simulink model "main_state_v2"  (R2021b)
settings: Solver=VariableStepAuto  StartTime=0.0  StopTime=10.0  RelTol=1e-3
settings Model: Creator=nose  LastModifiedBy=nose

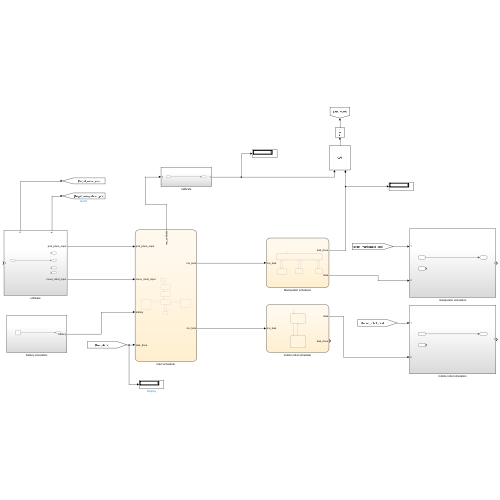
[thumbnail: Simulink's stored preview of the top-level diagram]
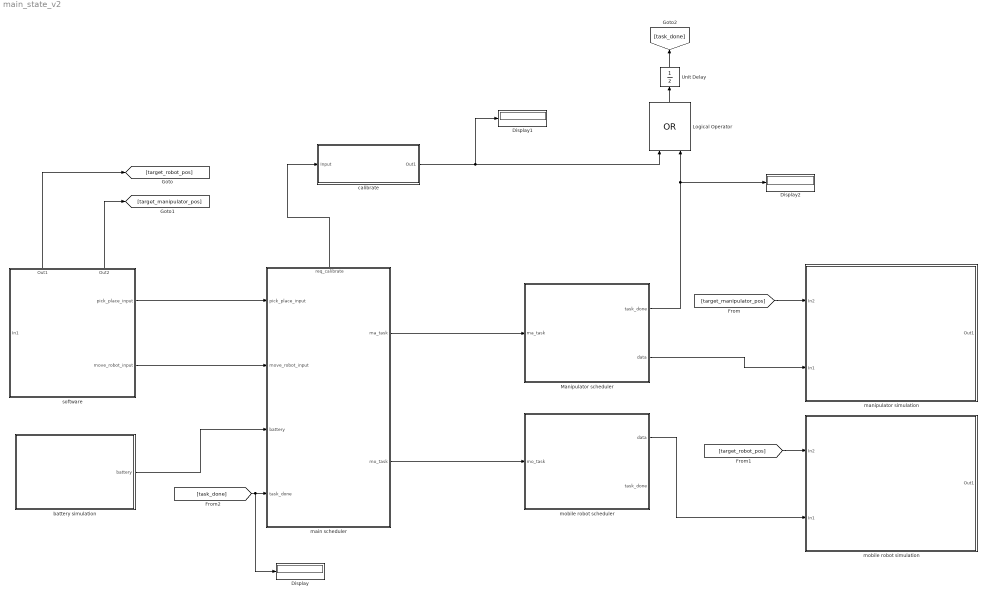
== system main_state_v2 ==
  Display : Display
  Display1 : Display
  Display2 : Display
  Logical Operator : Logic  Operator=OR  AllPortsSameDT=off  OutDataTypeStr=boolean
  Manipulator scheduler : Stateflow chart  TreatAsAtomicUnit=on
  Unit Delay : UnitDelay  SampleTime=-1  HasFrameUpgradeWarning=on
  battery simulation : Subsystem
  calibrate : Subsystem
  main scheduler : Stateflow chart  TreatAsAtomicUnit=on
      settings: PortSchema="{\"entries\":[{\"content\":{\"sides\":[{\"content\":{\"connectorIds\":[\"In1\",\"In4\",\"In2\",\"In3\"]},\"type\":\"ConnectorPlacement.EquallySpacedRectSide\",\"uuid\":\"f5729231-57ab-4499-afbb-6a74bae65d7c\"},{\"content\":{\"connectorIds\":[\"Out2\",\"Out3\"],\"side\":\"RIGHT\"},\"type\":\"ConnectorPlacement.EquallySpacedRectSide\",\"uuid\":\"4bea4fd3-2ca8-4b6f-84e5-251c5021326e\"},{\"content\":{\"connectorIds\":[\"Out1\"],\"side\":\"TOP\"},\"type\":\"ConnectorPlacement.EquallySpacedRectSide\",\"uuid\":\"ba10ffa7-10a0-4e15-a1ab-c6799962567e\"}]},\"type\":\"ConnectorPlacement.EquallySpacedConnector\",\"uuid\":\"fd2ab94f-7982-477b-afda-6ae5ba1f9b27\"}],\"packageUris\":[\"http://schema.mathworks.com/mf0/Connector/R2020b\"],\"version\":\"1.0\"}"
  manipulator simulation : Subsystem
  mobile robot scheduler : Stateflow chart  TreatAsAtomicUnit=on
  mobile robot simulation : Subsystem
  software : Subsystem
      settings: PortSchema="{\"entries\":[{\"content\":{\"sides\":[{\"content\":{\"connectorIds\":[\"In1\"]},\"type\":\"ConnectorPlacement.EquallySpacedRectSide\",\"uuid\":\"68df7bb9-dda6-4834-bc86-6120b81067a6\"},{\"content\":{\"connectorIds\":[\"Out1\",\"Out2\"],\"side\":\"RIGHT\"},\"type\":\"ConnectorPlacement.EquallySpacedRectSide\",\"uuid\":\"97ff30f2-6e8d-41db-be67-1bd246f3902f\"},{\"content\":{\"connectorIds\":[\"Out3\",\"Out4\"],\"side\":\"TOP\"},\"type\":\"ConnectorPlacement.EquallySpacedRectSide\",\"uuid\":\"a9bfe2b4-c08a-4e3f-8415-e43960abb484\"}]},\"type\":\"ConnectorPlacement.EquallySpacedConnector\",\"uuid\":\"6637d52b-a5d0-4863-9f23-94af3600c1a1\"}],\"packageUris\":[\"http://schema.mathworks.com/mf0/Connector/R2020b\"],\"version\":\"1.0\"}"
  wires:
  main scheduler/2(ma_task) -> Manipulator scheduler/1(ma_task)
  main scheduler/3(mo_task) -> mobile robot scheduler/1(mo_task)
  main scheduler/1(req_calibrate) -> calibrate/1(Input)
  battery simulation/1(battery) -> main scheduler/2(battery)
  software/1(pick_place_input) -> main scheduler/1(pick_place_input)
  software/2(move_robot_input) -> main scheduler/4(move_robot_input)
  software/3(Out1) -> [target_robot_pos]
  software/4(Out2) -> [target_manipulator_pos]
  [target_manipulator_pos] -> manipulator simulation/1(In2)
  [target_robot_pos] -> mobile robot simulation/1(In2)
  Manipulator scheduler/2(data) -> manipulator simulation/2(In1)
  mobile robot scheduler/1(data) -> mobile robot simulation/2(In1)
  [task_done] -> Display/1, main scheduler/3(task_done)
  calibrate/1(Out1) -> Display1/1, Logical Operator/1
  Manipulator scheduler/1(task_done) -> Display2/1, Logical Operator/2
  Logical Operator/1 -> Unit Delay/1
  Unit Delay/1 -> [task_done]

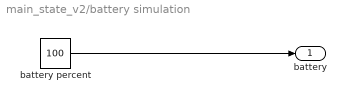
== system main_state_v2/battery simulation ==
  battery percent : Constant  Value=100
  battery : Outport
  wires:
  battery percent/1 -> battery/1

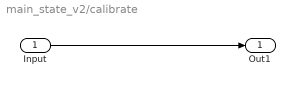
== system main_state_v2/calibrate ==
  Input : Inport
  Out1 : Outport
  wires:
  Input/1 -> Out1/1

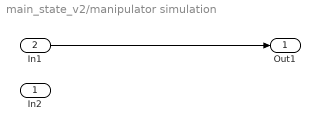
== system main_state_v2/manipulator simulation ==
  In2 : Inport
  In1 : Inport  Port=2
  Out1 : Outport
  wires:
  In1/1 -> Out1/1

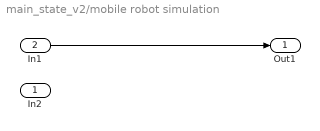
== system main_state_v2/mobile robot simulation ==
  In2 : Inport
  In1 : Inport  Port=2
  Out1 : Outport
  wires:
  In1/1 -> Out1/1

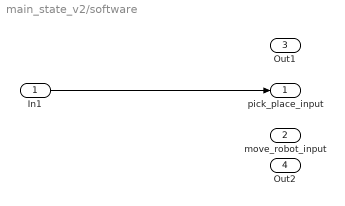
== system main_state_v2/software ==
  In1 : Inport
  pick_place_input : Outport
  move_robot_input : Outport  Port=2
  Out1 : Outport  Port=3
  Out2 : Outport  Port=4
  wires:
  In1/1 -> pick_place_input/1

== stateflow chart main_state_v2/mobile robot scheduler ==
  state idle
    en:
    task_done = false;
  state move
    en:
    data = 1;
  (default) -> idle
  idle -> move : [mo_task == 1]
  move -> idle : {task_done = true;}
  data: mo_task input; data output; task_done output

== stateflow chart main_state_v2/Manipulator scheduler ==
  state idle
    en:
    task_done = false;
  state home
    en:
    task_done = true;
    data = 1;
  state pick
    en:
    data = 2;
  state place
    en:
    data = 3;
  (default) -> idle
  idle -> home [order 1] : [ma_task == 1]
  home -> idle
  idle -> pick [order 2] : [ma_task == 2]
  pick -> idle
  idle -> place [order 3] : [ma_task == 3]
  place -> idle
  data: task_done output; ma_task input; data output

== stateflow chart main_state_v2/main scheduler ==
  state Start
    en:
    ma_task = 0;
    mo_task = 0;
  state calibrate
    en:
    req_calibrate = 1;
    exit:
    req_calibrate = 0;
  state home_arm
    en:
    ma_task = 1;
  state pick_place
    en:
    if(pick_place_input == 1)
    ma_task = 2;
    elseif(pick_place_input == 2)
    ma_task = 3;
    end
  state ready
    en:
    ma_task = 0;
    mo_task = 0;
  state move_robot
    en:
    mo_task = 1;
  note: pick_place_input:
      | 0 -> no input
      | 1 -> pick
      | 2 -> place
  state go_charge
  (default) -> Start
  Start -> calibrate
  calibrate -> home_arm : [task_done == true]
  home_arm -> ready : [task_done == true]
  ready -> pick_place [order 2] : [pick_place_input > 0]
  ready -> move_robot [order 3] : [move_robot_input == 1]
  pick_place -> ready
  move_robot -> ready
  ready -> go_charge [order 1] : [battery < 10]
  go_charge -> ready : [task_done == true]
  data: pick_place_input input; battery input; req_calibrate output; task_done input; move_robot_input input; ma_task output; mo_task output
